simulink model "match"  (R2024a)
settings: Solver=VariableStepAuto  StartTime=0.0  StopTime=60  RelTol=1e-3
values from neighbouring files (symbols this model uses):
  beta0 = 1    [data.m]
  Map_CD = ReshapeMatrix(data0,data4,data8,flag_CD)    [data.m]
  Map_CL = ReshapeMatrix(data0,data4,data8,flag_CL)    [data.m]
undefined symbols (not defined in the file or in its folder): EmptyWeight, FullWeight, Pa, Sc, VMax
libraries: simulink x6, aerolibatmos2 x6
settings Model: Creator=10335  LastModifiedBy=10335

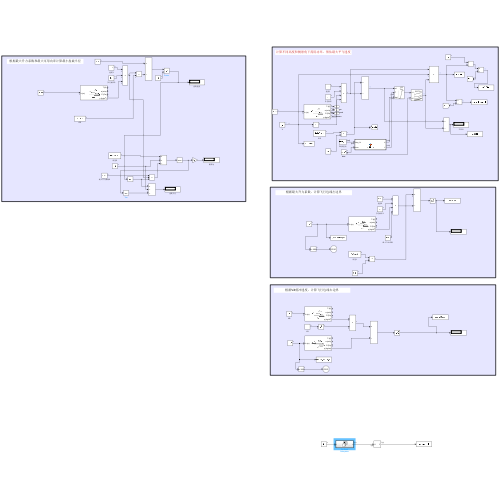
[thumbnail: Simulink's stored preview of the top-level diagram]
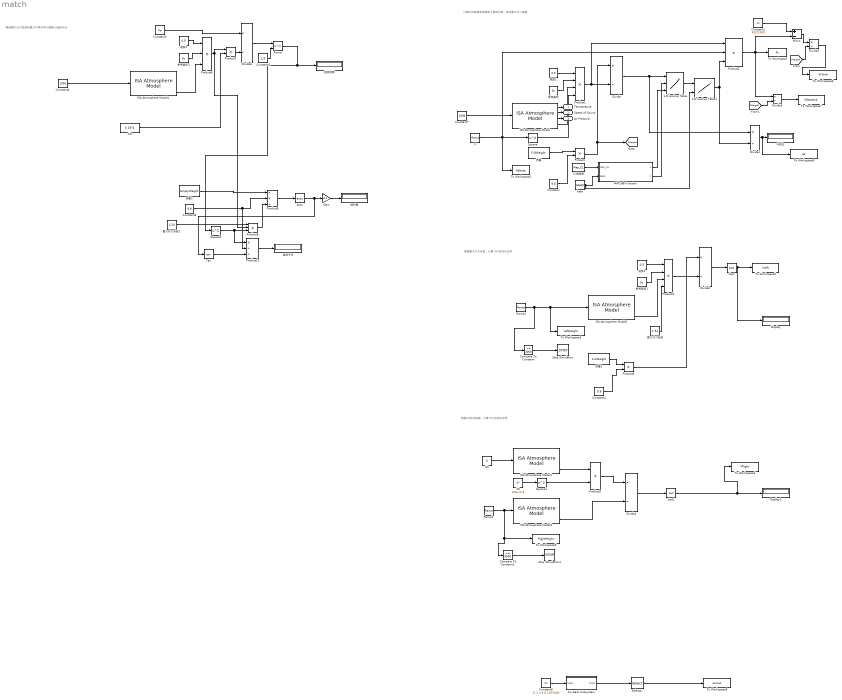
== system match ==
  note: 根据最大升力系数，计算飞行包线左边界
  note: 根据Vd俯冲速度，计算飞行包线右边界
  note: 根据最大升力系数和最大可用功率计算最小盘旋半径
  note: 计算不同高度和侧滑角下需用功率，预估最大平飞速度
  1-D Lookup Table : Lookup_n-D  NumberOfTableDimensions=1  BreakpointsForDimension1Source=Input port  BreakpointsForDimension1=[-5:5]  TableSource=Input port  Table=tanh([-5:5])  InternalRulePriority=Speed  RndMeth=Simplest
      settings: InputPortMap=u0,p221,p5
  1-D Lookup Table1 : Lookup_n-D  BreakpointsForDimension1=[0 4 8]  BreakpointsForDimension2=[0 5 10 15 20 25]  Table=Map_CD  InternalRulePriority=Speed  RndMeth=Simplest
      settings: InputPortMap=u0,u1
  Acos : Trigonometry  Operator=acos
  CD : Constant  Value=0.1974
  CL插值表 : Constant  Value=Map_CL
  Compare To Constant : simulink/Logic and Bit Operations/Compare To Constant  relop=>=  const=3000  OutDataTypeStr=boolean
  Compare To Constant1 : simulink/Logic and Bit Operations/Compare To Constant  relop=>=  const=3000  OutDataTypeStr=boolean
  Constant : Constant  Value=9.8
  Constant1 : Constant  Value=432*1000
  Constant2 : Constant  Value=9.8
  Constant3 : Constant  Value=Pa
  Constant4 : Constant  Value=1000
  Constant5 : Constant  Value=1/3
  Constant6 : Constant  Value=9.8
  Constant7 : Constant  Value=1000
  Constant8 : Constant  Value=[1 2 4 6 8 10]*1000
  Display : Display
  Display1 : Display
  Divide{,1..6} (7 alike) : Product  Inputs=*/
  For Each Subsystem : Subsystem  TreatAsAtomicUnit=on
  Gain : Gain  Gain=57.3
  H0 : Constant  Value=0
  ISA Atmosphere Model{,1..4} (5 alike) : aerolibatmos2/ISA Atmosphere Model  useExtended=off  action=Warning  custom=off  viscosityOut=off  g=9.80665  gamma=1.4  R=287.0531  L=0.0065  h_trop=11000  h_strat=20000  rho0=1.225  P0=101325  T0=288.15  h0=0  S=110.4  Tref=273.15  muref=1.716e-5
  MATLAB Function : MATLAB Function  TreatAsAtomicUnit=on
  Minus : Sum  Inputs=+-
  Power : Math  Operator=pow
  Product{,4..5,7} (4 alike) : Product
  Product1 : Product  Inputs=4
  Product10 : Product  Inputs=*//
  Product2 : Product  Inputs=3
  Product3 : Product  Inputs=4
  Product6 : Product  Inputs=3
  Product8 : Product  Inputs=**/
  Product9 : Product  Inputs=3
  Ramp1 : simulink/Sources/Ramp  slope=200  start=0  InitialOutput=0
  Ramp2 : simulink/Sources/Ramp  slope=200  start=0  InitialOutput=0
  Selector : Selector  InputPortWidth=6  IndexOptions=Index vector (dialog)  Indices=[1]  OutputSizes=1
  Sqrt : Sqrt
  Sqrt1 : Sqrt
  Square : Math  Operator=square
  Square1 : Math  Operator=square
  Square2 : Math  Operator=square
  Stop Simulation : Stop
  Stop Simulation1 : Stop
  Tan : Trigonometry  Operator=tan
  To Workspace : ToWorkspace  VariableName=Pc  SaveFormat=Structure  SampleTime=-1
  To Workspace1 : ToWorkspace  VariableName=Velocity  SaveFormat=Structure  SampleTime=-1
  To Workspace2 : ToWorkspace  VariableName=VLeft  SaveFormat=Structure  SampleTime=-1
  To Workspace3 : ToWorkspace  VariableName=LeftHeight  SaveFormat=Structure  SampleTime=-1
  To Workspace4 : ToWorkspace  VariableName=VRight  SaveFormat=Structure  SampleTime=-1
  To Workspace5 : ToWorkspace  VariableName=RightHeight  SaveFormat=Structure  SampleTime=-1
  To Workspace6 : ToWorkspace  VariableName=VClimb  SaveFormat=Structure  SampleTime=-1
  To Workspace7 : ToWorkspace  VariableName=VDescend  SaveFormat=Structure  SampleTime=-1
  To Workspace8 : ToWorkspace  VariableName=simout  SaveFormat=Timeseries  SampleTime=-1
  To Workspace9 : ToWorkspace  VariableName=LD  SaveFormat=Structure  SampleTime=-1
  V : simulink/Sources/Ramp  slope=1  start=0  InitialOutput=45
  V0 : Constant  Value=VMax/3.6
  beta : Constant  Value=beta0
  倾斜角 : Display
  升阻比 : Display
  参考面积 : Constant  Value=Sc
  参考面积1 : Constant  Value=Sc
  参考面积2 : Constant  Value=Sc
  最大升力系数 : Constant  Value=1.54
  最大升力系数2 : Constant  Value=1.54
  盘旋半径 : Display
  盘旋速度 : Display
  质量 : Constant  Value=FullWeight
  质量1 : Constant  Value=FullWeight
  质量2 : Constant  Value=EmptyWeight
  速度1 : Constant  Value=0.5
  速度2 : Constant  Value=0.5
  速度3 : Constant  Value=0.5
  Temperature : Outport
  Speed of Sound : Outport  Port=2
  Air Pressure : Outport  Port=3
  wires:
  Divide2/1 -> Sqrt/1
  Product4/1 -> Divide2/1
  Product3/1 -> Divide2/2
  参考面积1/1 -> Product3/2
  最大升力系数/1 -> Product3/4
  速度2/1 -> Product3/1
  ISA Atmosphere Model2/4 -> Product3/3
  Ramp1/1 -> Compare To Constant/1, To Workspace3/1, ISA Atmosphere Model2/1
  质量1/1 -> Product4/1
  Constant2/1 -> Product4/2
  Sqrt/1 -> Display/1, To Workspace2/1
  Sqrt1/1 -> To Workspace4/1, Display1/1
  H0/1 -> ISA Atmosphere Model1/1
  Divide4/1 -> Sqrt1/1
  V0/1 -> Square1/1
  ISA Atmosphere Model1/4 -> Product5/1
  Square1/1 -> Product5/2
  Ramp2/1 -> Compare To Constant1/1, To Workspace5/1, ISA Atmosphere Model3/1
  Product5/1 -> Divide4/1
  ISA Atmosphere Model3/4 -> Divide4/2
  Constant4/1 -> ISA Atmosphere Model4/1
  速度3/1 -> Product6/1
  参考面积2/1 -> Product6/2
  Constant3/1 -> Divide6/1
  ISA Atmosphere Model4/4 -> Product6/3
  Compare To Constant/1 -> Stop Simulation/1
  Compare To Constant1/1 -> Stop Simulation1/1
  最大升力系数2/1 -> Product9/1
  Constant5/1 -> Power/2
  Power/1 -> Square2/1, 盘旋速度/1
  Product7/1 -> Divide6/2
  Product6/1 -> Product7/1, Product9/2
  CD/1 -> Product7/2
  质量2/1 -> Product8/1
  Constant6/1 -> Product10/2, Product8/2
  Square2/1 -> Product10/1, Product9/3
  Product9/1 -> Product8/3
  Product8/1 -> Acos/1
  Acos/1 -> Tan/1, Gain/1
  Gain/1 -> 倾斜角/1
  Divide6/1 -> Power/1
  Tan/1 -> Product10/3
  Product10/1 -> 盘旋半径/1
  参考面积/1 -> Product1/2
  MATLAB Function/2(Y) -> 1-D Lookup Table/2
  MATLAB Function/1(X) -> 1-D Lookup Table/3
  [Weight] -> Divide3/2
  ISA Atmosphere Model/3 -> Air Pressure/1
  Divide3/1 -> To Workspace6/1
  Constant1/1 -> Minus/1
  ISA Atmosphere Model/1 -> Temperature/1
  Divide1/1 -> To Workspace9/1, 升阻比/1
  Constant7/1 -> ISA Atmosphere Model/1
  Product/1 -> Divide/1, [Weight]
  CL插值表/1 -> MATLAB Function/1(Map_CL)
  质量/1 -> Product/1
  Minus/1 -> Divide3/1
  Product1/1 -> Product2/1, Divide/2
  速度1/1 -> Product1/1
  beta/1 -> 1-D Lookup Table1/2, MATLAB Function/2(beta)
  [Weight] -> Divide5/2
  1-D Lookup Table/1 -> 1-D Lookup Table1/1
  Product2/1 -> Divide5/1, Minus/2, To Workspace/1
  Constant/1 -> Product/2
  ISA Atmosphere Model/4 -> Product1/3
  Divide/1 -> Divide1/1, 1-D Lookup Table/1
  V/1 -> Product2/2, To Workspace1/1, Square/1
  ISA Atmosphere Model/2 -> Speed of Sound/1
  Divide5/1 -> To Workspace7/1
  1-D Lookup Table1/1 -> Product2/3, Divide1/2
  Square/1 -> Product1/4
  Constant8/1 -> For Each Subsystem/1(Input)
  For Each Subsystem/1(Out1) -> Selector/1
  Selector/1 -> To Workspace8/1

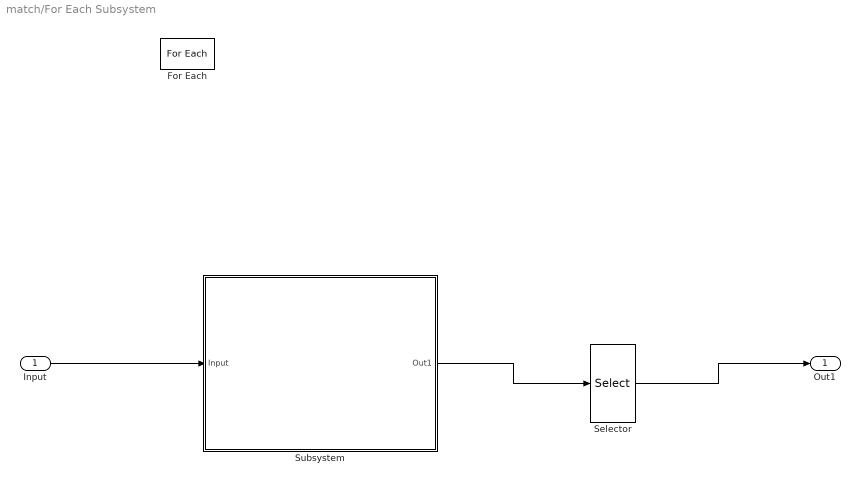
== system match/For Each Subsystem ==
  Input : Inport  Partition=on  PartitionDimension=2  PartitionWidth=1  PartitionOffset=0
  For Each : ForEach  DisableCoverage=on
  Selector : Selector  InputPortWidth=6  IndexOptions=Index vector (dialog)  Indices=[1]  OutputSizes=1
  Subsystem : Subsystem
  Out1 : Outport  ConcatenationDimension=1
  wires:
  Input/1 -> Subsystem/1(Input)
  Subsystem/1(Out1) -> Selector/1
  Selector/1 -> Out1/1

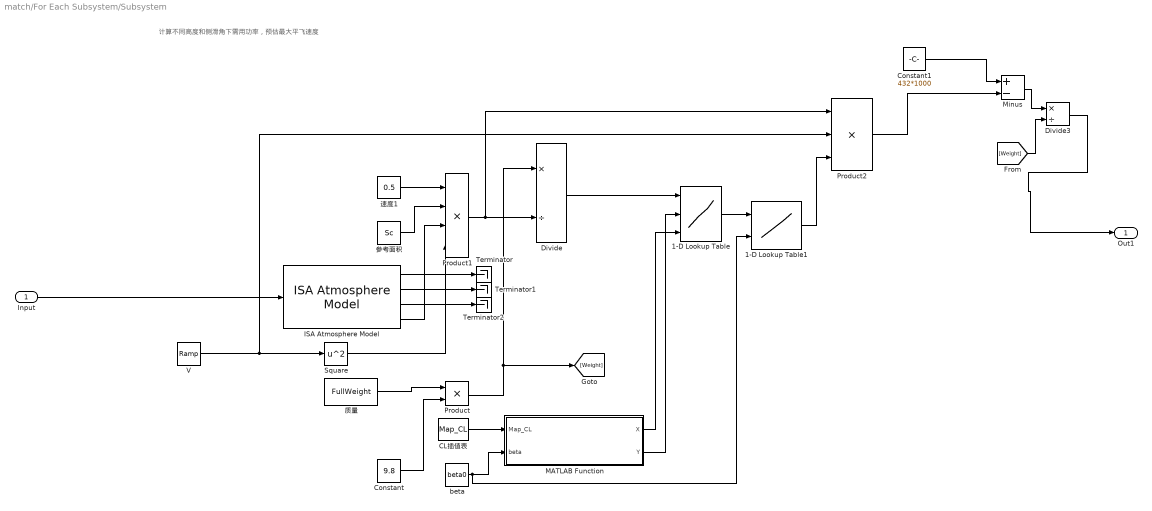
== system match/For Each Subsystem/Subsystem ==
  note: 计算不同高度和侧滑角下需用功率，预估最大平飞速度
  Input : Inport
  1-D Lookup Table : Lookup_n-D  NumberOfTableDimensions=1  BreakpointsForDimension1Source=Input port  BreakpointsForDimension1=[-5:5]  TableSource=Input port  Table=tanh([-5:5])  InternalRulePriority=Speed  RndMeth=Simplest
      settings: InputPortMap=u0,p221,p5
  1-D Lookup Table1 : Lookup_n-D  BreakpointsForDimension1=[0 4 8]  BreakpointsForDimension2=[0 5 10 15 20 25]  Table=Map_CD  InternalRulePriority=Speed  RndMeth=Simplest
      settings: InputPortMap=u0,u1
  CL插值表 : Constant  Value=Map_CL
  Constant : Constant  Value=9.8
  Constant1 : Constant  Value=432*1000
  Divide : Product  Inputs=*/
  Divide3 : Product  Inputs=*/
  ISA Atmosphere Model : aerolibatmos2/ISA Atmosphere Model  useExtended=off  action=Warning  custom=off  viscosityOut=off  g=9.80665  gamma=1.4  R=287.0531  L=0.0065  h_trop=11000  h_strat=20000  rho0=1.225  P0=101325  T0=288.15  h0=0  S=110.4  Tref=273.15  muref=1.716e-5
  MATLAB Function : MATLAB Function  TreatAsAtomicUnit=on
  Minus : Sum  Inputs=+-
  Product : Product
  Product1 : Product  Inputs=4
  Product2 : Product  Inputs=3
  Square : Math  Operator=square
  Terminator : Terminator
  Terminator1 : Terminator
  Terminator2 : Terminator
  V : simulink/Sources/Ramp  slope=1  start=0  InitialOutput=45
  beta : Constant  Value=beta0
  参考面积 : Constant  Value=Sc
  质量 : Constant  Value=FullWeight
  速度1 : Constant  Value=0.5
  Out1 : Outport
  wires:
  Divide3/1 -> Out1/1
  V/1 -> Product2/2, Square/1
  Divide/1 -> 1-D Lookup Table/1
  Product2/1 -> Minus/2
  Constant/1 -> Product/2
  beta/1 -> 1-D Lookup Table1/2, MATLAB Function/2(beta)
  Product1/1 -> Product2/1, Divide/2
  速度1/1 -> Product1/1
  Square/1 -> Product1/4
  Minus/1 -> Divide3/1
  质量/1 -> Product/1
  1-D Lookup Table/1 -> 1-D Lookup Table1/1
  MATLAB Function/1(X) -> 1-D Lookup Table/3
  ISA Atmosphere Model/4 -> Product1/3
  Input/1 -> ISA Atmosphere Model/1
  CL插值表/1 -> MATLAB Function/1(Map_CL)
  Product/1 -> Divide/1, [Weight]
  1-D Lookup Table1/1 -> Product2/3
  MATLAB Function/2(Y) -> 1-D Lookup Table/2
  Constant1/1 -> Minus/1
  ISA Atmosphere Model/3 -> Terminator2/1
  参考面积/1 -> Product1/2
  ISA Atmosphere Model/1 -> Terminator/1
  [Weight] -> Divide3/2
  ISA Atmosphere Model/2 -> Terminator1/1

== matlab function match/MATLAB Function ==
  data: Map_CL input; X output; beta input; Y output

function [X,Y]=InvMatrix(Map_CL,beta)
X=Map_CL(1:3,beta)';
Y=[0 4 8];

== matlab function match/For Each Subsystem/Subsystem/MATLAB Function ==
  data: Map_CL input; X output; beta input; Y output

function [X,Y]=InvMatrix(Map_CL,beta)
X=Map_CL(1:3,beta)';
Y=[0 4 8];
